simulink model "hip1"  (R2020a)
settings: Solver=VariableStepAuto  StartTime=0.0  StopTime=10.0  RelTol=1e-3
undefined symbols (not defined in the file or in its folder): freq
settings Model: Creator=david  LastModifiedBy=david

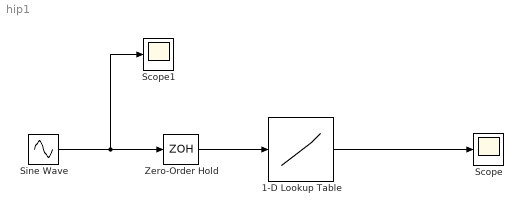
== system hip1 ==
  1-D Lookup Table : Lookup_n-D  NumberOfTableDimensions=1  BreakpointsForDimension1=[-5:5]  Table=tanh([-5:5])  InternalRulePriority=Speed  RndMeth=Simplest  InputSameDT=on
  Scope : Scope
  Scope1 : Scope
  Sine Wave : Sin  Frequency=freq  SampleTime=1/30000
  Zero-Order Hold : ZeroOrderHold  SampleTime=1/30000
  wires:
  Sine Wave/1 -> Scope1/1, Zero-Order Hold/1
  Zero-Order Hold/1 -> 1-D Lookup Table/1
  1-D Lookup Table/1 -> Scope/1
